simulink model "Labex2si3"  (R2021b)
settings: Solver=VariableStepAuto  StartTime=0.0  StopTime=120.0  RelTol=1e-3
settings Model: Creator=User  LastModifiedBy=User

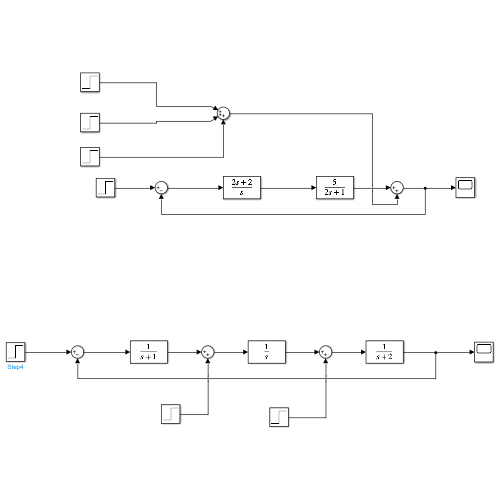
[thumbnail: Simulink's stored preview of the top-level diagram]
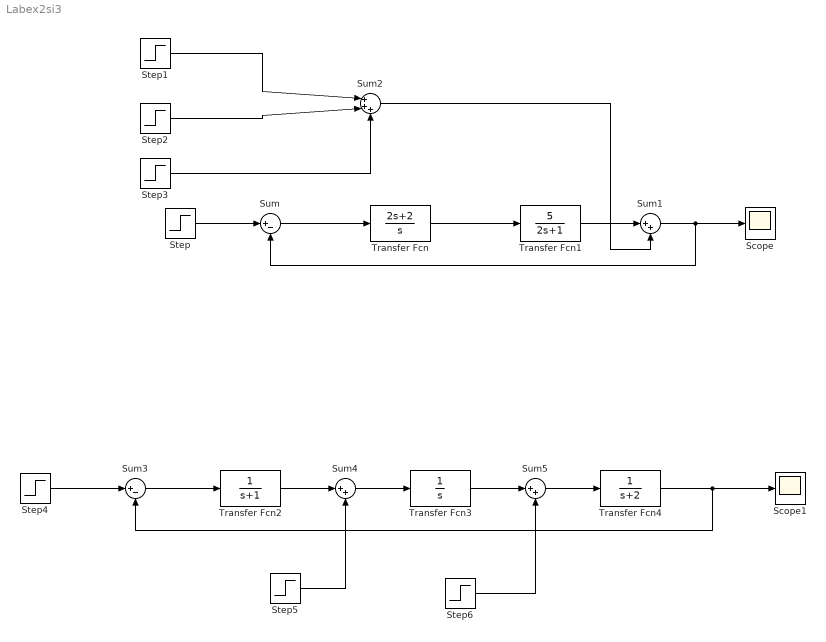
== system Labex2si3 ==
  Scope : Scope
  Scope1 : Scope
  Step : Step  SampleTime=0
  Step1 : Step  Time=10  After=0.2  SampleTime=0
  Step2 : Step  Time=20  After=0.1  SampleTime=0
  Step3 : Step  Time=30  After=0.1  SampleTime=0
  Step4 : Step  SampleTime=0
  Step5 : Step  Time=40  SampleTime=0
  Step6 : Step  Time=80  SampleTime=0
  Sum : Sum  Inputs=|+-
  Sum1 : Sum  Inputs=|++
  Sum2 : Sum  Inputs=|+++
  Sum3 : Sum  Inputs=|+-
  Sum4 : Sum  Inputs=|++
  Sum5 : Sum  Inputs=|++
  Transfer Fcn : TransferFcn  Numerator=[2 2]  Denominator=[1 0]
  Transfer Fcn1 : TransferFcn  Numerator=[5]  Denominator=[2 1]
  Transfer Fcn2 : TransferFcn  Denominator=[1 1]
  Transfer Fcn3 : TransferFcn  Denominator=[1 0]
  Transfer Fcn4 : TransferFcn  Denominator=[1 2]
  wires:
  Sum/1 -> Transfer Fcn/1
  Transfer Fcn/1 -> Transfer Fcn1/1
  Transfer Fcn1/1 -> Sum1/1
  Sum1/1 -> Sum/2, Scope/1
  Step/1 -> Sum/1
  Step1/1 -> Sum2/1
  Step2/1 -> Sum2/2
  Step3/1 -> Sum2/3
  Sum2/1 -> Sum1/2
  Step4/1 -> Sum3/1
  Sum3/1 -> Transfer Fcn2/1
  Transfer Fcn2/1 -> Sum4/1
  Sum4/1 -> Transfer Fcn3/1
  Transfer Fcn3/1 -> Sum5/1
  Sum5/1 -> Transfer Fcn4/1
  Transfer Fcn4/1 -> Sum3/2, Scope1/1
  Step5/1 -> Sum4/2
  Step6/1 -> Sum5/2
